simulink model "pp_forward"  (R2022b)
settings: Solver=VariableStepAuto  StartTime=0.0  StopTime=250  RelTol=1e-3
values from neighbouring files (symbols this model uses):
  cx = 0:0.1:120    [cungz_ref_01.m]
libraries: Solver_SF x1, simulink x1
settings Model: Creator=admin  LastModifiedBy=admin

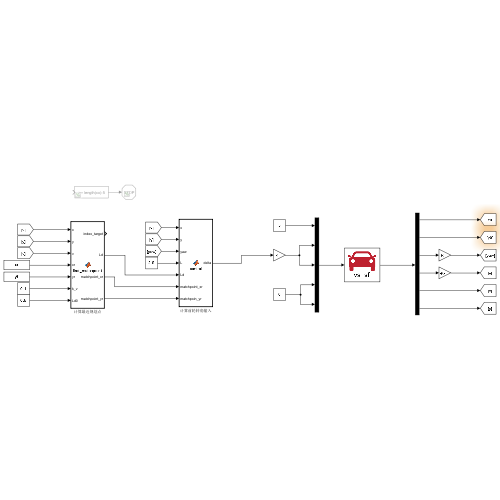
[thumbnail: Simulink's stored preview of the top-level diagram]
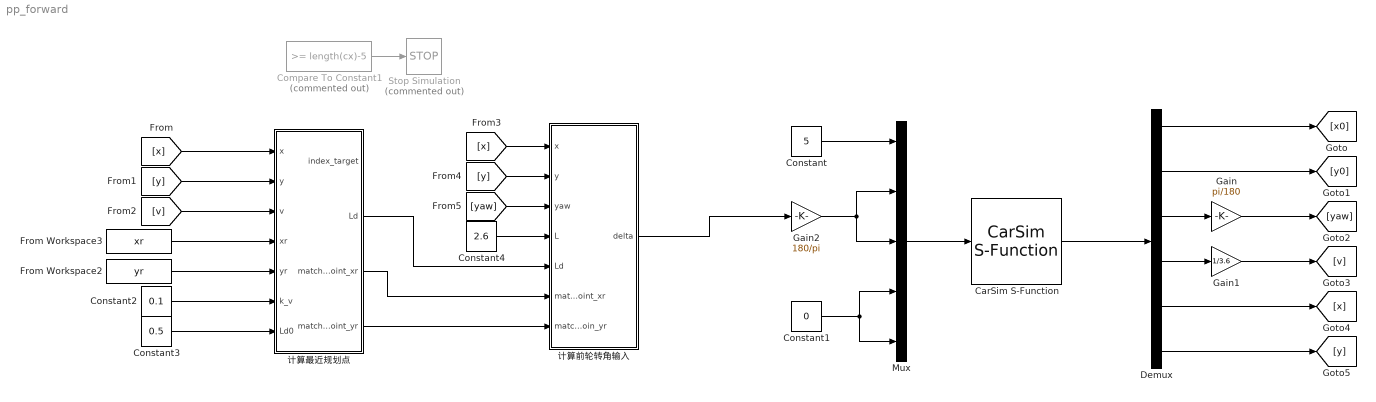
== system pp_forward ==
  CarSim S-Function : Solver_SF/CarSim S-Function  Priority=1  SIMFILE=simfile.sim  Run_RTs=off  vs_state_ind=Run  StopMode_ind=Vehicle Model
  Compare To Constant1 : simulink/Logic and Bit Operations/Compare To Constant  Commented=on  relop=>=  const=length(cx)-5  OutDataTypeStr=boolean
  Constant : Constant  Value=5
  Constant1 : Constant  Value=0
  Constant2 : Constant  Value=0.1
  Constant3 : Constant  Value=0.5
  Constant4 : Constant  Value=2.6
  Demux : Demux  Outputs=6
  From Workspace2 : FromWorkspace  VariableName=yr
  From Workspace3 : FromWorkspace  VariableName=xr
  Gain : Gain  Gain=pi/180
  Gain1 : Gain  Gain=1/3.6
  Gain2 : Gain  Gain=180/pi
  Mux : Mux  Inputs=5
  Stop Simulation : Stop  Commented=on
  计算前轮转角输入 : MATLAB Function  TreatAsAtomicUnit=on
  计算最近规划点 : MATLAB Function  TreatAsAtomicUnit=on
  wires:
  Demux/1 -> [x0]
  Demux/2 -> [y0]
  Demux/3 -> Gain/1
  Gain/1 -> [yaw]
  Demux/4 -> Gain1/1
  Gain1/1 -> [v]
  Demux/5 -> [x]
  Mux/1 -> CarSim S-Function/1
  Constant/1 -> Mux/1
  Gain2/1 -> Mux/2, Mux/3
  计算前轮转角输入/1(delta) -> Gain2/1
  Constant1/1 -> Mux/5, Mux/4
  [x] -> 计算最近规划点/1(x)
  [y] -> 计算最近规划点/2(y)
  [v] -> 计算最近规划点/3(v)
  From Workspace2/1 -> 计算最近规划点/5(yr)
  Constant2/1 -> 计算最近规划点/6(k_v)
  Constant3/1 -> 计算最近规划点/7(Ld0)
  Compare To Constant1/1 -> Stop Simulation/1
  [x] -> 计算前轮转角输入/1(x)
  [y] -> 计算前轮转角输入/2(y)
  [yaw] -> 计算前轮转角输入/3(yaw)
  计算最近规划点/2(Ld) -> 计算前轮转角输入/5(Ld)
  Constant4/1 -> 计算前轮转角输入/4(L)
  计算最近规划点/3(matchpoint_xr) -> 计算前轮转角输入/6(matchpoint_xr)
  计算最近规划点/4(matchpoint_yr) -> 计算前轮转角输入/7(matchpoin_yr)
  CarSim S-Function/1 -> Demux/1
  Demux/6 -> [y]
  From Workspace3/1 -> 计算最近规划点/4(xr)

== matlab function pp_forward/计算前轮转角输入 ==
  data: x input; delta output; y input; yaw input; L input; Ld input; matchpoint_xr input; matchpoin_yr input
function delta = control(x,y,yaw,L,Ld,matchpoint_xr,matchpoin_yr)
    %计算车轴与匹配点连线之间的夹角alpha
    alpha = atan2((matchpoin_yr - y), (matchpoint_xr - x)) - yaw;
    %计算前轮转角
    delta = atan2(2*L*sin(alpha), Ld);
    %限制前轮转角大小
%     if delta < -pi/3
%         delta = -pi/3;
%     elseif delta > pi/3
%         delta = pi/3;
%     end
    if delta < -pi/3
        delta = -pi/3;
    end
    if delta > pi/3
        delta = pi/3;
    end
end

== matlab function pp_forward/计算最近规划点 ==
  data: x input; index_target output; y input; v input; xr input; yr input; k_v input; Ld0 input; Ld output; matchpoint_xr output; matchpoint_yr output
function [index_target, Ld, matchpoint_xr, matchpoint_yr] = find_matchpoint(x,y,v,xr,yr,k_v,Ld0)
    total_point = length(xr);
    index_min = 0;
    distance_min = (xr(1) - x)^2 + (yr(1) -y)^2;
    for i=1:total_point
        distance = (xr(i) - x)^2 + (yr(i) -y)^2;    %这里不用加根号函数，因为只是找最近的点，平方也无所谓
        if distance < distance_min
            distance_min = distance;
            index_min = i;      %最近规划点的索引值
        end
    end
    
    %设置初始累加距离
    L_step = 0;
    Ld = k_v*v + Ld0;   %前视距离Ld
    
    if index_min < 1
        index_min = 1;
    end

    while L_step < Ld && index_min < total_point
        L_step = sqrt((xr(index_min+1)-xr(index_min))^2 + (yr(index_min+1)-yr(index_min))^2) + L_step;
        index_min = index_min + 1;
    end

    %匹配点索引值
    index_target = index_min;
    %获取匹配点坐标
    matchpoint_xr = xr(index_target);
    matchpoint_yr = yr(index_target);
end
